simulink model "P702_NI_SoftECU"  (R2019a)
settings: Solver=ode1  StartTime=0.0  StopTime=Inf  FixedStep=0.001  RelTol=1e-3  EnableMultiTasking=on
PreLoadFcn:
  | run '.\VeriStand_BlockSet\NIVeriStandAddPaths.m'
undefined symbols (not defined in the file or in its folder): magnitude
libraries: simulink x83, simulink_extras x1
(part 72 of 76)

== system P702_NI_SoftECU/Output/Subsystem1/CAN_Signal/GWM/Other_GWMTx/Climate_Cntrl_Data_2_FD1 ==
  in_port : Inport
  ApaSwtch_D_RqDrv : Terminator
  ApaSwtch_No_Cnt : Terminator
  CabnAmb_Te_Actl : Terminator
  CamraDefog_B_Actl : Terminator
  ClimtThrmlLoad_No_Actl : Terminator
  EcoMde_D_RqDrv : Terminator
  HvacAir_Flw_Est : Terminator
  HvacBlwrFront_D_Stat : Terminator
  HvacBlwrRear_D_Stat : Terminator
  HvacRec_Pc_Est : Terminator
  HvacRemoteStrt_N_Rq : Terminator
  TwHlGrdAsst_B_RqTrn : Terminator
  bus_selector : BusSelector  OutputSignals=ApaSwtch_D_RqDrv,ApaSwtch_No_Cnt,CabnAmb_Te_Actl,CamraDefog_B_Actl,ClimtThrmlLoad_No_Actl,EcoMde_D_RqDrv,HvacAir_Flw_Est,HvacBlwrFront_D_Stat,HvacBlwrRear_D_Stat,HvacRec_Pc_Est,HvacRemoteStrt_N_Rq,TwHlGrdAsst_B_RqTrn
  wires:
  in_port/1 -> bus_selector/1  "Subsystem1"
  bus_selector/1 -> ApaSwtch_D_RqDrv/1  "<ApaSwtch_D_RqDrv>"
  bus_selector/2 -> ApaSwtch_No_Cnt/1  "<ApaSwtch_No_Cnt>"
  bus_selector/3 -> CabnAmb_Te_Actl/1  "<CabnAmb_Te_Actl>"
  bus_selector/4 -> CamraDefog_B_Actl/1  "<CamraDefog_B_Actl>"
  bus_selector/5 -> ClimtThrmlLoad_No_Actl/1  "<ClimtThrmlLoad_No_Actl>"
  bus_selector/6 -> EcoMde_D_RqDrv/1  "<EcoMde_D_RqDrv>"
  bus_selector/7 -> HvacAir_Flw_Est/1  "<HvacAir_Flw_Est>"
  bus_selector/8 -> HvacBlwrFront_D_Stat/1  "<HvacBlwrFront_D_Stat>"
  bus_selector/9 -> HvacBlwrRear_D_Stat/1  "<HvacBlwrRear_D_Stat>"
  bus_selector/10 -> HvacRec_Pc_Est/1  "<HvacRec_Pc_Est>"
  bus_selector/11 -> HvacRemoteStrt_N_Rq/1  "<HvacRemoteStrt_N_Rq>"
  bus_selector/12 -> TwHlGrdAsst_B_RqTrn/1  "<TwHlGrdAsst_B_RqTrn>"

== system P702_NI_SoftECU/Output/Subsystem1/CAN_Signal/GWM/Other_GWMTx/Climate_Control_Data_FD1 ==
  in_port : Inport
  AutoHoldSwtch_D_Stat : Terminator
  CamraFrntBttn_D_Stat : Terminator
  CamraRearBttn_D_Stat : Terminator
  DrvSlipCtlMde_B_Rq : Terminator
  EcoInhbt_B_RqHvac : Terminator
  GlvBoxRleas_No_Actl : Terminator
  LpdbAuxBlwr_B_Rq : Terminator
  LpdbDfrstFlOn_B_Rq : Terminator
  LpdbDfrstFrOn_B_Rq : Terminator
  LpdbDfrstRearOn_B_Rq : Terminator
  LpdbHeatWiprPrk_B_Rq : Terminator
  LpdbPtc1_B_Rq : Terminator
  LpdbPtc2_B_Rq : Terminator
  LpdbPtc3_B_Rq : Terminator
  MirrorHeatOn_B_Rq : Terminator
  Outside_Air_Temp_Stat : Terminator
  PrkAidSwtch_D_RqDrv : Terminator
  PrkAidSwtch_No_Cnt : Terminator
  Remote_Start_QuietMode : Terminator
  SteWhlHeat_D_Rq : Terminator
  TrailCtlSwtch_B_Stat : Terminator
  bus_selector : BusSelector  OutputSignals=AutoHoldSwtch_D_Stat,CamraFrntBttn_D_Stat,CamraRearBttn_D_Stat,DrvSlipCtlMde_B_Rq,EcoInhbt_B_RqHvac,GlvBoxRleas_No_Actl,LpdbAuxBlwr_B_Rq,LpdbDfrstFlOn_B_Rq,LpdbDfrstFrOn_B_Rq,LpdbDfrstRearOn_B_Rq,LpdbHeatWiprPrk_B_Rq,LpdbPtc1_B_Rq,LpdbPtc2_B_Rq,LpdbPtc3_B_Rq,MirrorHeatOn_B_Rq,Outside_Air_Temp_Stat,PrkAidSwtch_D_RqDrv,PrkAidSwtch_No_Cnt,Remote_Start_QuietMode,SteWhlHeat_D_Rq,TrailCtlSwtch_B_Stat
  wires:
  in_port/1 -> bus_selector/1  "Subsystem1"
  bus_selector/1 -> AutoHoldSwtch_D_Stat/1  "<AutoHoldSwtch_D_Stat>"
  bus_selector/2 -> CamraFrntBttn_D_Stat/1  "<CamraFrntBttn_D_Stat>"
  bus_selector/3 -> CamraRearBttn_D_Stat/1  "<CamraRearBttn_D_Stat>"
  bus_selector/4 -> DrvSlipCtlMde_B_Rq/1  "<DrvSlipCtlMde_B_Rq>"
  bus_selector/5 -> EcoInhbt_B_RqHvac/1  "<EcoInhbt_B_RqHvac>"
  bus_selector/6 -> GlvBoxRleas_No_Actl/1  "<GlvBoxRleas_No_Actl>"
  bus_selector/7 -> LpdbAuxBlwr_B_Rq/1  "<LpdbAuxBlwr_B_Rq>"
  bus_selector/8 -> LpdbDfrstFlOn_B_Rq/1  "<LpdbDfrstFlOn_B_Rq>"
  bus_selector/9 -> LpdbDfrstFrOn_B_Rq/1  "<LpdbDfrstFrOn_B_Rq>"
  bus_selector/10 -> LpdbDfrstRearOn_B_Rq/1  "<LpdbDfrstRearOn_B_Rq>"
  bus_selector/11 -> LpdbHeatWiprPrk_B_Rq/1  "<LpdbHeatWiprPrk_B_Rq>"
  bus_selector/12 -> LpdbPtc1_B_Rq/1  "<LpdbPtc1_B_Rq>"
  bus_selector/13 -> LpdbPtc2_B_Rq/1  "<LpdbPtc2_B_Rq>"
  bus_selector/14 -> LpdbPtc3_B_Rq/1  "<LpdbPtc3_B_Rq>"
  bus_selector/15 -> MirrorHeatOn_B_Rq/1  "<MirrorHeatOn_B_Rq>"
  bus_selector/16 -> Outside_Air_Temp_Stat/1  "<Outside_Air_Temp_Stat>"
  bus_selector/17 -> PrkAidSwtch_D_RqDrv/1  "<PrkAidSwtch_D_RqDrv>"
  bus_selector/18 -> PrkAidSwtch_No_Cnt/1  "<PrkAidSwtch_No_Cnt>"
  bus_selector/19 -> Remote_Start_QuietMode/1  "<Remote_Start_QuietMode>"
  bus_selector/20 -> SteWhlHeat_D_Rq/1  "<SteWhlHeat_D_Rq>"
  bus_selector/21 -> TrailCtlSwtch_B_Stat/1  "<TrailCtlSwtch_B_Stat>"

== system P702_NI_SoftECU/Output/Subsystem1/CAN_Signal/GWM/Other_GWMTx/Cluster_Info1_FD1 ==
  in_port : Inport
  AccDeny_B_RqIpc : Terminator
  AccEnbl_B_RqDrv : Terminator
  BulbChkActv_B_Stat : Terminator
  DrvPerfMde_D_Rq : Terminator
  DrvSlipCtlMde_B_Rq2 : Terminator
  DrvSlipCtlMde_D_Rq : Terminator
  EmgcyCallAsstMykey_Rq : Terminator
  EngIdlShutDown_B_RqDrv : Terminator
  EngOilLife_B_RqReset : Terminator
  Fda_B_Stat : Terminator
  FrostWarn_D_Stat : Terminator
  HsaMde_D_Rq : Terminator
  KeyTypeChngMykey_D_Rq : Terminator
  LscmbbStat_B_Actl : Terminator
  ManRgen_D_Rq : Terminator
  MetricActvTe_B_Actl : Terminator
  MetricActv_B_Actl : Terminator
  NtrlTowMdeEnbl_B_RqDrv : Terminator
  OdometerMasterValue : Terminator
  ParkDetect_Stat : Terminator
  Power_Liftgate_Mode_Cmd : Terminator
  PrkLckCtlEnbl_D_RqIpc : Terminator
  PtDrvMde_D_Rq : Terminator
  ReducedGuard_D_Rq : Terminator
  StopStrtDrvMde_D_RqMnu : Terminator
  TRAILER_BRAKE_CONFIG : Terminator
  TRLR_SWAY_CONFIG_CMD : Terminator
  TrlrBrkMde_D_Rq : Terminator
  bus_selector : BusSelector  OutputSignals=AccDeny_B_RqIpc,AccEnbl_B_RqDrv,BulbChkActv_B_Stat,DrvPerfMde_D_Rq,DrvSlipCtlMde_B_Rq2,DrvSlipCtlMde_D_Rq,EmgcyCallAsstMykey_Rq,EngIdlShutDown_B_RqDrv,EngOilLife_B_RqReset,Fda_B_Stat,FrostWarn_D_Stat,HsaMde_D_Rq,KeyTypeChngMykey_D_Rq,LscmbbStat_B_Actl,ManRgen_D_Rq,MetricActvTe_B_Actl,MetricActv_B_Actl,NtrlTowMdeEnbl_B_RqDrv,OdometerMasterValue,ParkDetect_Stat,Power_Liftgate_Mode_Cmd,PrkLckCtlEnbl_D_RqIpc,PtDrvMde_D_Rq,ReducedGuard_D_Rq,StopStrtDrvMde_D_RqMnu,TRAILER_BRAKE_CONFIG,TRLR_SWAY_CONFIG_CMD,TrlrBrkMde_D_Rq,ePRNDL_MODE
  ePRNDL_MODE : Terminator
  wires:
  in_port/1 -> bus_selector/1  "Subsystem1"
  bus_selector/1 -> AccDeny_B_RqIpc/1  "<AccDeny_B_RqIpc>"
  bus_selector/2 -> AccEnbl_B_RqDrv/1  "<AccEnbl_B_RqDrv>"
  bus_selector/3 -> BulbChkActv_B_Stat/1  "<BulbChkActv_B_Stat>"
  bus_selector/4 -> DrvPerfMde_D_Rq/1  "<DrvPerfMde_D_Rq>"
  bus_selector/5 -> DrvSlipCtlMde_B_Rq2/1  "<DrvSlipCtlMde_B_Rq2>"
  bus_selector/6 -> DrvSlipCtlMde_D_Rq/1  "<DrvSlipCtlMde_D_Rq>"
  bus_selector/7 -> EmgcyCallAsstMykey_Rq/1  "<EmgcyCallAsstMykey_Rq>"
  bus_selector/8 -> EngIdlShutDown_B_RqDrv/1  "<EngIdlShutDown_B_RqDrv>"
  bus_selector/9 -> EngOilLife_B_RqReset/1  "<EngOilLife_B_RqReset>"
  bus_selector/10 -> Fda_B_Stat/1  "<Fda_B_Stat>"
  bus_selector/11 -> FrostWarn_D_Stat/1  "<FrostWarn_D_Stat>"
  bus_selector/12 -> HsaMde_D_Rq/1  "<HsaMde_D_Rq>"
  bus_selector/13 -> KeyTypeChngMykey_D_Rq/1  "<KeyTypeChngMykey_D_Rq>"
  bus_selector/14 -> LscmbbStat_B_Actl/1  "<LscmbbStat_B_Actl>"
  bus_selector/15 -> ManRgen_D_Rq/1  "<ManRgen_D_Rq>"
  bus_selector/16 -> MetricActvTe_B_Actl/1  "<MetricActvTe_B_Actl>"
  bus_selector/17 -> MetricActv_B_Actl/1  "<MetricActv_B_Actl>"
  bus_selector/18 -> NtrlTowMdeEnbl_B_RqDrv/1  "<NtrlTowMdeEnbl_B_RqDrv>"
  bus_selector/19 -> OdometerMasterValue/1  "<OdometerMasterValue>"
  bus_selector/20 -> ParkDetect_Stat/1  "<ParkDetect_Stat>"
  bus_selector/21 -> Power_Liftgate_Mode_Cmd/1  "<Power_Liftgate_Mode_Cmd>"
  bus_selector/22 -> PrkLckCtlEnbl_D_RqIpc/1  "<PrkLckCtlEnbl_D_RqIpc>"
  bus_selector/23 -> PtDrvMde_D_Rq/1  "<PtDrvMde_D_Rq>"
  bus_selector/24 -> ReducedGuard_D_Rq/1  "<ReducedGuard_D_Rq>"
  bus_selector/25 -> StopStrtDrvMde_D_RqMnu/1  "<StopStrtDrvMde_D_RqMnu>"
  bus_selector/26 -> TRAILER_BRAKE_CONFIG/1  "<TRAILER_BRAKE_CONFIG>"
  bus_selector/27 -> TRLR_SWAY_CONFIG_CMD/1  "<TRLR_SWAY_CONFIG_CMD>"
  bus_selector/28 -> TrlrBrkMde_D_Rq/1  "<TrlrBrkMde_D_Rq>"
  bus_selector/29 -> ePRNDL_MODE/1  "<ePRNDL_MODE>"

== system P702_NI_SoftECU/Output/Subsystem1/CAN_Signal/GWM/Other_GWMTx/Cluster_Info_3_FD1 ==
  in_port : Inport
  AutoRgen_D_Rq : Terminator
  DISPLAY_SPEED_OFFSET : Terminator
  DISPLAY_SPEED_SCALING : Terminator
  DrvSlipCtlMde_B_RqMyKey : Terminator
  FUEL_SENSOR_NUM : Terminator
  FuelLvlActvSide_No_Raw : Terminator
  FuelLvlPssvSide_No_Raw : Terminator
  FuelLvlWarn_D_Actl : Terminator
  FuelLvl_Pc_Dsply : Terminator
  FuelSecndActv_B_Actl : Terminator
  OdoTripRx_B_Actl : Terminator
  Veh_V_CompLimMx : Terminator
  W2S_LAMP_OK : Terminator
  bus_selector : BusSelector  OutputSignals=AutoRgen_D_Rq,DISPLAY_SPEED_OFFSET,DISPLAY_SPEED_SCALING,DrvSlipCtlMde_B_RqMyKey,FUEL_SENSOR_NUM,FuelLvlActvSide_No_Raw,FuelLvlPssvSide_No_Raw,FuelLvlWarn_D_Actl,FuelLvl_Pc_Dsply,FuelSecndActv_B_Actl,OdoTripRx_B_Actl,Veh_V_CompLimMx,W2S_LAMP_OK
  wires:
  in_port/1 -> bus_selector/1  "Subsystem1"
  bus_selector/1 -> AutoRgen_D_Rq/1  "<AutoRgen_D_Rq>"
  bus_selector/2 -> DISPLAY_SPEED_OFFSET/1  "<DISPLAY_SPEED_OFFSET>"
  bus_selector/3 -> DISPLAY_SPEED_SCALING/1  "<DISPLAY_SPEED_SCALING>"
  bus_selector/4 -> DrvSlipCtlMde_B_RqMyKey/1  "<DrvSlipCtlMde_B_RqMyKey>"
  bus_selector/5 -> FUEL_SENSOR_NUM/1  "<FUEL_SENSOR_NUM>"
  bus_selector/6 -> FuelLvlActvSide_No_Raw/1  "<FuelLvlActvSide_No_Raw>"
  bus_selector/7 -> FuelLvlPssvSide_No_Raw/1  "<FuelLvlPssvSide_No_Raw>"
  bus_selector/8 -> FuelLvlWarn_D_Actl/1  "<FuelLvlWarn_D_Actl>"
  bus_selector/9 -> FuelLvl_Pc_Dsply/1  "<FuelLvl_Pc_Dsply>"
  bus_selector/10 -> FuelSecndActv_B_Actl/1  "<FuelSecndActv_B_Actl>"
  bus_selector/11 -> OdoTripRx_B_Actl/1  "<OdoTripRx_B_Actl>"
  bus_selector/12 -> Veh_V_CompLimMx/1  "<Veh_V_CompLimMx>"
  bus_selector/13 -> W2S_LAMP_OK/1  "<W2S_LAMP_OK>"

== system P702_NI_SoftECU/Output/Subsystem1/CAN_Signal/GWM/Other_GWMTx/Cluster_Lighting_Rq_FD1 ==
  in_port : Inport
  IsaOffst_D_Rq : Terminator
  SlMde_D_Rq : Terminator
  bus_selector : BusSelector  OutputSignals=IsaOffst_D_Rq,SlMde_D_Rq
  wires:
  in_port/1 -> bus_selector/1  "Subsystem1"
  bus_selector/1 -> IsaOffst_D_Rq/1  "<IsaOffst_D_Rq>"
  bus_selector/2 -> SlMde_D_Rq/1  "<SlMde_D_Rq>"

== system P702_NI_SoftECU/Output/Subsystem1/CAN_Signal/GWM/Other_GWMTx/Compressor_Req_FD1 ==
  in_port : Inport
  ClimtCoolRear_B_Rq : Terminator
  ClimtCool_D_Rq : Terminator
  ClimtDeltaLoad_Pw_Actl : Terminator
  ClimtHeatRear_D_Rq : Terminator
  ClimtHeat_D_Rq : Terminator
  ClimtPw_B_Rq : Terminator
  HtrCorePump_B_Rq : Terminator
  HvacAirCond_B_Rq : Terminator
  HvacEvap_Te_Actl : Terminator
  HvacEvap_Te_Offst : Terminator
  HvacEvap_Te_Rq : Terminator
  HvacHtrCore_Te_Rq : Terminator
  SnowPlowMde_B_Enbl : Terminator
  StopStrtDrvMde_B_RqBtn : Terminator
  WndwFrontHeat_B_Stat : Terminator
  bus_selector : BusSelector  OutputSignals=ClimtCoolRear_B_Rq,ClimtCool_D_Rq,ClimtDeltaLoad_Pw_Actl,ClimtHeatRear_D_Rq,ClimtHeat_D_Rq,ClimtPw_B_Rq,HtrCorePump_B_Rq,HvacAirCond_B_Rq,HvacEvap_Te_Actl,HvacEvap_Te_Offst,HvacEvap_Te_Rq,HvacHtrCore_Te_Rq,SnowPlowMde_B_Enbl,StopStrtDrvMde_B_RqBtn,WndwFrontHeat_B_Stat
  wires:
  in_port/1 -> bus_selector/1  "Subsystem1"
  bus_selector/1 -> ClimtCoolRear_B_Rq/1  "<ClimtCoolRear_B_Rq>"
  bus_selector/2 -> ClimtCool_D_Rq/1  "<ClimtCool_D_Rq>"
  bus_selector/3 -> ClimtDeltaLoad_Pw_Actl/1  "<ClimtDeltaLoad_Pw_Actl>"
  bus_selector/4 -> ClimtHeatRear_D_Rq/1  "<ClimtHeatRear_D_Rq>"
  bus_selector/5 -> ClimtHeat_D_Rq/1  "<ClimtHeat_D_Rq>"
  bus_selector/6 -> ClimtPw_B_Rq/1  "<ClimtPw_B_Rq>"
  bus_selector/7 -> HtrCorePump_B_Rq/1  "<HtrCorePump_B_Rq>"
  bus_selector/8 -> HvacAirCond_B_Rq/1  "<HvacAirCond_B_Rq>"
  bus_selector/9 -> HvacEvap_Te_Actl/1  "<HvacEvap_Te_Actl>"
  bus_selector/10 -> HvacEvap_Te_Offst/1  "<HvacEvap_Te_Offst>"
  bus_selector/11 -> HvacEvap_Te_Rq/1  "<HvacEvap_Te_Rq>"
  bus_selector/12 -> HvacHtrCore_Te_Rq/1  "<HvacHtrCore_Te_Rq>"
  bus_selector/13 -> SnowPlowMde_B_Enbl/1  "<SnowPlowMde_B_Enbl>"
  bus_selector/14 -> StopStrtDrvMde_B_RqBtn/1  "<StopStrtDrvMde_B_RqBtn>"
  bus_selector/15 -> WndwFrontHeat_B_Stat/1  "<WndwFrontHeat_B_Stat>"

== system P702_NI_SoftECU/Output/Subsystem1/CAN_Signal/GWM/Other_GWMTx/CruiseCtrl_Strg_Data_FD1 ==
  in_port : Inport
  AccButtnGapDecPress2 : Terminator
  AccButtnGapIncPress2 : Terminator
  AccButtnGpTogglePress2 : Terminator
  ActvFrontSteLck_D_Stat : Terminator
  ActvFrontSteMsgTxt_D_Rq : Terminator
  AslButtnOnOffCnclPres2 : Terminator
  AslButtnOnOffPress2 : Terminator
  CcAslButtnCnclPress2 : Terminator
  CcAslButtnCnclResPres2 : Terminator
  CcAslButtnDeny_B_Actl2 : Terminator
  CcAslButtnIndxDecPres2 : Terminator
  CcAslButtnIndxIncPres2 : Terminator
  CcAslButtnOffCnclPres2 : Terminator
  CcAslButtnOnOffCncl2 : Terminator
  CcAslButtnOnPress2 : Terminator
  CcAslButtnResDecPress2 : Terminator
  CcAslButtnResIncPress2 : Terminator
  CcAslButtnSetDecPress2 : Terminator
  CcAslButtnSetIncPress2 : Terminator
  CcAslButtnSetPress2 : Terminator
  CcAsllButtnResPress2 : Terminator
  CcButtnOffPress2 : Terminator
  CcButtnOnOffCnclPress2 : Terminator
  CcButtnOnOffPress2 : Terminator
  CcButtnOnPress2 : Terminator
  SelDrvMdeAdptSte_D_Stat : Terminator
  TjaButtnOnOffPress2 : Terminator
  bus_selector : BusSelector  OutputSignals=AccButtnGapDecPress2,AccButtnGapIncPress2,AccButtnGpTogglePress2,ActvFrontSteLck_D_Stat,ActvFrontSteMsgTxt_D_Rq,AslButtnOnOffCnclPres2,AslButtnOnOffPress2,CcAslButtnCnclPress2,CcAslButtnCnclResPres2,CcAslButtnDeny_B_Actl2,CcAslButtnIndxDecPres2,CcAslButtnIndxIncPres2,CcAslButtnOffCnclPres2,CcAslButtnOnOffCncl2,CcAslButtnOnPress2,CcAslButtnResDecPress2,CcAslButtnResIncPress2,CcAslButtnSetDecPress2,CcAslButtnSetIncPress2,CcAslButtnSetPress2,CcAsllButtnResPress2,CcButtnOffPress2,CcButtnOnOffCnclPress2,CcButtnOnOffPress2,CcButtnOnPress2,SelDrvMdeAdptSte_D_Stat,TjaButtnOnOffPress2
  wires:
  in_port/1 -> bus_selector/1  "Subsystem1"
  bus_selector/1 -> AccButtnGapDecPress2/1  "<AccButtnGapDecPress2>"
  bus_selector/2 -> AccButtnGapIncPress2/1  "<AccButtnGapIncPress2>"
  bus_selector/3 -> AccButtnGpTogglePress2/1  "<AccButtnGpTogglePress2>"
  bus_selector/4 -> ActvFrontSteLck_D_Stat/1  "<ActvFrontSteLck_D_Stat>"
  bus_selector/5 -> ActvFrontSteMsgTxt_D_Rq/1  "<ActvFrontSteMsgTxt_D_Rq>"
  bus_selector/6 -> AslButtnOnOffCnclPres2/1  "<AslButtnOnOffCnclPres2>"
  bus_selector/7 -> AslButtnOnOffPress2/1  "<AslButtnOnOffPress2>"
  bus_selector/8 -> CcAslButtnCnclPress2/1  "<CcAslButtnCnclPress2>"
  bus_selector/9 -> CcAslButtnCnclResPres2/1  "<CcAslButtnCnclResPres2>"
  bus_selector/10 -> CcAslButtnDeny_B_Actl2/1  "<CcAslButtnDeny_B_Actl2>"
  bus_selector/11 -> CcAslButtnIndxDecPres2/1  "<CcAslButtnIndxDecPres2>"
  bus_selector/12 -> CcAslButtnIndxIncPres2/1  "<CcAslButtnIndxIncPres2>"
  bus_selector/13 -> CcAslButtnOffCnclPres2/1  "<CcAslButtnOffCnclPres2>"
  bus_selector/14 -> CcAslButtnOnOffCncl2/1  "<CcAslButtnOnOffCncl2>"
  bus_selector/15 -> CcAslButtnOnPress2/1  "<CcAslButtnOnPress2>"
  bus_selector/16 -> CcAslButtnResDecPress2/1  "<CcAslButtnResDecPress2>"
  bus_selector/17 -> CcAslButtnResIncPress2/1  "<CcAslButtnResIncPress2>"
  bus_selector/18 -> CcAslButtnSetDecPress2/1  "<CcAslButtnSetDecPress2>"
  bus_selector/19 -> CcAslButtnSetIncPress2/1  "<CcAslButtnSetIncPress2>"
  bus_selector/20 -> CcAslButtnSetPress2/1  "<CcAslButtnSetPress2>"
  bus_selector/21 -> CcAsllButtnResPress2/1  "<CcAsllButtnResPress2>"
  bus_selector/22 -> CcButtnOffPress2/1  "<CcButtnOffPress2>"
  bus_selector/23 -> CcButtnOnOffCnclPress2/1  "<CcButtnOnOffCnclPress2>"
  bus_selector/24 -> CcButtnOnOffPress2/1  "<CcButtnOnOffPress2>"
  bus_selector/25 -> CcButtnOnPress2/1  "<CcButtnOnPress2>"
  bus_selector/26 -> SelDrvMdeAdptSte_D_Stat/1  "<SelDrvMdeAdptSte_D_Stat>"
  bus_selector/27 -> TjaButtnOnOffPress2/1  "<TjaButtnOnOffPress2>"

== system P702_NI_SoftECU/Output/Subsystem1/CAN_Signal/GWM/Other_GWMTx/DCACA_Data1_FD1 ==
  in_port : Inport
  CoolFanDcac_D_Rq : Terminator
  DcacClntFlw_D_Rq : Terminator
  DcacPlugPrsnt_B_Stat : Terminator
  DcacRdy_D_Stat : Terminator
  bus_selector : BusSelector  OutputSignals=CoolFanDcac_D_Rq,DcacClntFlw_D_Rq,DcacPlugPrsnt_B_Stat,DcacRdy_D_Stat
  wires:
  in_port/1 -> bus_selector/1  "Subsystem1"
  bus_selector/1 -> CoolFanDcac_D_Rq/1  "<CoolFanDcac_D_Rq>"
  bus_selector/2 -> DcacClntFlw_D_Rq/1  "<DcacClntFlw_D_Rq>"
  bus_selector/3 -> DcacPlugPrsnt_B_Stat/1  "<DcacPlugPrsnt_B_Stat>"
  bus_selector/4 -> DcacRdy_D_Stat/1  "<DcacRdy_D_Stat>"

== system P702_NI_SoftECU/Output/Subsystem1/CAN_Signal/GWM/Other_GWMTx/DCACA_Data2_FD1 ==
  in_port : Inport
  DcacIn_I_Actl : Terminator
  DcacIn_U_Actl : Terminator
  Dcac_Te_Actl : Terminator
  bus_selector : BusSelector  OutputSignals=DcacIn_I_Actl,DcacIn_U_Actl,Dcac_Te_Actl
  wires:
  in_port/1 -> bus_selector/1  "Subsystem1"
  bus_selector/1 -> DcacIn_I_Actl/1  "<DcacIn_I_Actl>"
  bus_selector/2 -> DcacIn_U_Actl/1  "<DcacIn_U_Actl>"
  bus_selector/3 -> Dcac_Te_Actl/1  "<Dcac_Te_Actl>"

== system P702_NI_SoftECU/Output/Subsystem1/CAN_Signal/GWM/Other_GWMTx/DCACA_Data3_FD1 ==
  in_port : Inport
  DcacIn_Pw_Mx : Terminator
  DcacOut1_Pw_Actl : Terminator
  DcacOut2_Pw_Actl : Terminator
  DcacOut_Pw_Mx : Terminator
  bus_selector : BusSelector  OutputSignals=DcacIn_Pw_Mx,DcacOut1_Pw_Actl,DcacOut2_Pw_Actl,DcacOut_Pw_Mx
  wires:
  in_port/1 -> bus_selector/1  "Subsystem1"
  bus_selector/1 -> DcacIn_Pw_Mx/1  "<DcacIn_Pw_Mx>"
  bus_selector/2 -> DcacOut1_Pw_Actl/1  "<DcacOut1_Pw_Actl>"
  bus_selector/3 -> DcacOut2_Pw_Actl/1  "<DcacOut2_Pw_Actl>"
  bus_selector/4 -> DcacOut_Pw_Mx/1  "<DcacOut_Pw_Mx>"

== system P702_NI_SoftECU/Output/Subsystem1/CAN_Signal/GWM/Other_GWMTx/DifferentialCtrlData_1_FD1 ==
  in_port : Inport
  RearDiffLck_Tq_Actl2 : Terminator
  bus_selector : BusSelector  OutputSignals=RearDiffLck_Tq_Actl2
  wires:
  in_port/1 -> bus_selector/1  "Subsystem1"
  bus_selector/1 -> RearDiffLck_Tq_Actl2/1  "<RearDiffLck_Tq_Actl2>"

== system P702_NI_SoftECU/Output/Subsystem1/CAN_Signal/GWM/Other_GWMTx/Driver_Dr_Stat_FD1 ==
  in_port : Inport
  BLISLEDStatDriverSide : Terminator
  ChildLckFdbckRd_B_Stat : Terminator
  ChildLckPw_D_Rq : Terminator
  ChildLckPw_N_Cnt : Terminator
  Driver_Lock_Sw_Cnt : Terminator
  Driver_Lock_Sw_Stat : Terminator
  KeyCylSwDrvDr_D_Stat : Terminator
  RollCodeDrvDrKeyCyl : Terminator
  RvrseMirrorChime_B_Rq : Terminator
  WndwDrvSide_D_Stat : Terminator
  bus_selector : BusSelector  OutputSignals=BLISLEDStatDriverSide,ChildLckFdbckRd_B_Stat,ChildLckPw_D_Rq,ChildLckPw_N_Cnt,Driver_Lock_Sw_Cnt,Driver_Lock_Sw_Stat,KeyCylSwDrvDr_D_Stat,RollCodeDrvDrKeyCyl,RvrseMirrorChime_B_Rq,WndwDrvSide_D_Stat
  wires:
  in_port/1 -> bus_selector/1  "Subsystem1"
  bus_selector/1 -> BLISLEDStatDriverSide/1  "<BLISLEDStatDriverSide>"
  bus_selector/2 -> ChildLckFdbckRd_B_Stat/1  "<ChildLckFdbckRd_B_Stat>"
  bus_selector/3 -> ChildLckPw_D_Rq/1  "<ChildLckPw_D_Rq>"
  bus_selector/4 -> ChildLckPw_N_Cnt/1  "<ChildLckPw_N_Cnt>"
  bus_selector/5 -> Driver_Lock_Sw_Cnt/1  "<Driver_Lock_Sw_Cnt>"
  bus_selector/6 -> Driver_Lock_Sw_Stat/1  "<Driver_Lock_Sw_Stat>"
  bus_selector/7 -> KeyCylSwDrvDr_D_Stat/1  "<KeyCylSwDrvDr_D_Stat>"
  bus_selector/8 -> RollCodeDrvDrKeyCyl/1  "<RollCodeDrvDrKeyCyl>"
  bus_selector/9 -> RvrseMirrorChime_B_Rq/1  "<RvrseMirrorChime_B_Rq>"
  bus_selector/10 -> WndwDrvSide_D_Stat/1  "<WndwDrvSide_D_Stat>"

== system P702_NI_SoftECU/Output/Subsystem1/CAN_Signal/GWM/Other_GWMTx/Dsp_Request_Signals11_FD1 ==
  in_port : Inport
  ApaMdeStat_D_RqDrv : Terminator
  ApaSwtch_D_RqMnu : Terminator
  CamAutoTowbarZoom : Terminator
  CamraOvrlDyn_D_Rq : Terminator
  CamraOvrlStat_D_Rq : Terminator
  CamraViewSplit_B_Rq : Terminator
  CamraZoomMan_D_Rq : Terminator
  DistanceBarSetting : Terminator
  PrkAidSwtch_D_RqMnu : Terminator
  bus_selector : BusSelector  OutputSignals=ApaMdeStat_D_RqDrv,ApaSwtch_D_RqMnu,CamAutoTowbarZoom,CamraOvrlDyn_D_Rq,CamraOvrlStat_D_Rq,CamraViewSplit_B_Rq,CamraZoomMan_D_Rq,DistanceBarSetting,PrkAidSwtch_D_RqMnu
  wires:
  in_port/1 -> bus_selector/1  "Subsystem1"
  bus_selector/1 -> ApaMdeStat_D_RqDrv/1  "<ApaMdeStat_D_RqDrv>"
  bus_selector/2 -> ApaSwtch_D_RqMnu/1  "<ApaSwtch_D_RqMnu>"
  bus_selector/3 -> CamAutoTowbarZoom/1  "<CamAutoTowbarZoom>"
  bus_selector/4 -> CamraOvrlDyn_D_Rq/1  "<CamraOvrlDyn_D_Rq>"
  bus_selector/5 -> CamraOvrlStat_D_Rq/1  "<CamraOvrlStat_D_Rq>"
  bus_selector/6 -> CamraViewSplit_B_Rq/1  "<CamraViewSplit_B_Rq>"
  bus_selector/7 -> CamraZoomMan_D_Rq/1  "<CamraZoomMan_D_Rq>"
  bus_selector/8 -> DistanceBarSetting/1  "<DistanceBarSetting>"
  bus_selector/9 -> PrkAidSwtch_D_RqMnu/1  "<PrkAidSwtch_D_RqMnu>"

== system P702_NI_SoftECU/Output/Subsystem1/CAN_Signal/GWM/Other_GWMTx/ElecHorizon_Data1_FD1 ==
  in_port : Inport
  EhData1_No_Actl : Terminator
  bus_selector : BusSelector  OutputSignals=EhData1_No_Actl
  wires:
  in_port/1 -> bus_selector/1  "Subsystem1"
  bus_selector/1 -> EhData1_No_Actl/1  "<EhData1_No_Actl>"

== system P702_NI_SoftECU/Output/Subsystem1/CAN_Signal/GWM/Other_GWMTx/ElecHorizon_Data2_FD1 ==
  in_port : Inport
  EhData2_No_Actl : Terminator
  bus_selector : BusSelector  OutputSignals=EhData2_No_Actl
  wires:
  in_port/1 -> bus_selector/1  "Subsystem1"
  bus_selector/1 -> EhData2_No_Actl/1  "<EhData2_No_Actl>"

== system P702_NI_SoftECU/Output/Subsystem1/CAN_Signal/GWM/Other_GWMTx/FourByFourSwitchData_FD1 ==
  in_port : Inport
  AwdLck_D_RqDrv : Terminator
  AwdMde_D_RqDrv : Terminator
  DrvSlipCtlMde_B_Rq3 : Terminator
  HdcSwtchPos_B_Actl : Terminator
  HybMdeSwtch_B_Rq : Terminator
  RearDiffLck_D_RqDrv : Terminator
  TrailCtlSwtch_B_Stat3 : Terminator
  bus_selector : BusSelector  OutputSignals=AwdLck_D_RqDrv,AwdMde_D_RqDrv,DrvSlipCtlMde_B_Rq3,HdcSwtchPos_B_Actl,HybMdeSwtch_B_Rq,RearDiffLck_D_RqDrv,TrailCtlSwtch_B_Stat3
  wires:
  in_port/1 -> bus_selector/1  "Subsystem1"
  bus_selector/1 -> AwdLck_D_RqDrv/1  "<AwdLck_D_RqDrv>"
  bus_selector/2 -> AwdMde_D_RqDrv/1  "<AwdMde_D_RqDrv>"
  bus_selector/3 -> DrvSlipCtlMde_B_Rq3/1  "<DrvSlipCtlMde_B_Rq3>"
  bus_selector/4 -> HdcSwtchPos_B_Actl/1  "<HdcSwtchPos_B_Actl>"
  bus_selector/5 -> HybMdeSwtch_B_Rq/1  "<HybMdeSwtch_B_Rq>"
  bus_selector/6 -> RearDiffLck_D_RqDrv/1  "<RearDiffLck_D_RqDrv>"
  bus_selector/7 -> TrailCtlSwtch_B_Stat3/1  "<TrailCtlSwtch_B_Stat3>"

== system P702_NI_SoftECU/Output/Subsystem1/CAN_Signal/GWM/Other_GWMTx/Front_Distance_Req_FD1 ==
  in_port : Inport
  FdsmTrgCntr_B_Actl : Terminator
  FdsmTrgDist_L_Actl : Terminator
  FdsmTrgLeft_B_Actl : Terminator
  FdsmTrgRight_B_Actl : Terminator
  LscmbbBaSens_D_Rq : Terminator
  LscmbbBlck_B_Actl : Terminator
  LscmbbBrkDecel_A_Rq : Terminator
  LscmbbBrkDecel_B_Enbl : Terminator
  LscmbbBrkDecel_No_Cnt : Terminator
  LscmbbBrkDecel_No_Cs : Terminator
  LscmbbBrkPrchg_D_Rq : Terminator
  LscmbbDeny_B_Actl : Terminator
  LscmbbEngTqMn_B_Rq : Terminator
  LscmbbMsgTxt_D_Rq : Terminator
  LscmbbPostEvnt_B_Dsply : Terminator
  LscmbbSrvcRqd_B_Rq : Terminator
  WndwFrontHeat_B_Rq : Terminator
  bus_selector : BusSelector  OutputSignals=FdsmTrgCntr_B_Actl,FdsmTrgDist_L_Actl,FdsmTrgLeft_B_Actl,FdsmTrgRight_B_Actl,LscmbbBaSens_D_Rq,LscmbbBlck_B_Actl,LscmbbBrkDecel_A_Rq,LscmbbBrkDecel_B_Enbl,LscmbbBrkDecel_No_Cnt,LscmbbBrkDecel_No_Cs,LscmbbBrkPrchg_D_Rq,LscmbbDeny_B_Actl,LscmbbEngTqMn_B_Rq,LscmbbMsgTxt_D_Rq,LscmbbPostEvnt_B_Dsply,LscmbbSrvcRqd_B_Rq,WndwFrontHeat_B_Rq
  wires:
  in_port/1 -> bus_selector/1  "Subsystem1"
  bus_selector/1 -> FdsmTrgCntr_B_Actl/1  "<FdsmTrgCntr_B_Actl>"
  bus_selector/2 -> FdsmTrgDist_L_Actl/1  "<FdsmTrgDist_L_Actl>"
  bus_selector/3 -> FdsmTrgLeft_B_Actl/1  "<FdsmTrgLeft_B_Actl>"
  bus_selector/4 -> FdsmTrgRight_B_Actl/1  "<FdsmTrgRight_B_Actl>"
  bus_selector/5 -> LscmbbBaSens_D_Rq/1  "<LscmbbBaSens_D_Rq>"
  bus_selector/6 -> LscmbbBlck_B_Actl/1  "<LscmbbBlck_B_Actl>"
  bus_selector/7 -> LscmbbBrkDecel_A_Rq/1  "<LscmbbBrkDecel_A_Rq>"
  bus_selector/8 -> LscmbbBrkDecel_B_Enbl/1  "<LscmbbBrkDecel_B_Enbl>"
  bus_selector/9 -> LscmbbBrkDecel_No_Cnt/1  "<LscmbbBrkDecel_No_Cnt>"
  bus_selector/10 -> LscmbbBrkDecel_No_Cs/1  "<LscmbbBrkDecel_No_Cs>"
  bus_selector/11 -> LscmbbBrkPrchg_D_Rq/1  "<LscmbbBrkPrchg_D_Rq>"
  bus_selector/12 -> LscmbbDeny_B_Actl/1  "<LscmbbDeny_B_Actl>"
  bus_selector/13 -> LscmbbEngTqMn_B_Rq/1  "<LscmbbEngTqMn_B_Rq>"
  bus_selector/14 -> LscmbbMsgTxt_D_Rq/1  "<LscmbbMsgTxt_D_Rq>"
  bus_selector/15 -> LscmbbPostEvnt_B_Dsply/1  "<LscmbbPostEvnt_B_Dsply>"
  bus_selector/16 -> LscmbbSrvcRqd_B_Rq/1  "<LscmbbSrvcRqd_B_Rq>"
  bus_selector/17 -> WndwFrontHeat_B_Rq/1  "<WndwFrontHeat_B_Rq>"

== system P702_NI_SoftECU/Output/Subsystem1/CAN_Signal/GWM/Other_GWMTx/GGCC_Config_Mgmt_ID_1_FD1 ==
  in_port : Inport
  VehicleGGCCData : Terminator
  bus_selector : BusSelector  OutputSignals=VehicleGGCCData
  wires:
  in_port/1 -> bus_selector/1  "Subsystem1"
  bus_selector/1 -> VehicleGGCCData/1  "<VehicleGGCCData>"

== system P702_NI_SoftECU/Output/Subsystem1/CAN_Signal/GWM/Other_GWMTx/GWM_AutoSar_NetMgmt_FD1 ==
  in_port : Inport
  GWM_AutoSarNMControl : Terminator
  GWM_AutoSarNMNodeId : Terminator
  GWM_AutoSarNMReserved{1..4} (4 alike) : Terminator
  GWM_GWNMProxy : Terminator
  GWM_GWOnBoardTester : Terminator
  bus_selector : BusSelector  OutputSignals=GWM_AutoSarNMControl,GWM_AutoSarNMNodeId,GWM_AutoSarNMReserved1,GWM_AutoSarNMReserved2,GWM_AutoSarNMReserved3,GWM_AutoSarNMReserved4,GWM_GWNMProxy,GWM_GWOnBoardTester
  wires:
  in_port/1 -> bus_selector/1  "Subsystem1"
  bus_selector/1 -> GWM_AutoSarNMControl/1  "<GWM_AutoSarNMControl>"
  bus_selector/2 -> GWM_AutoSarNMNodeId/1  "<GWM_AutoSarNMNodeId>"
  bus_selector/3 -> GWM_AutoSarNMReserved1/1  "<GWM_AutoSarNMReserved1>"
  bus_selector/4 -> GWM_AutoSarNMReserved2/1  "<GWM_AutoSarNMReserved2>"
  bus_selector/5 -> GWM_AutoSarNMReserved3/1  "<GWM_AutoSarNMReserved3>"
  bus_selector/6 -> GWM_AutoSarNMReserved4/1  "<GWM_AutoSarNMReserved4>"
  bus_selector/7 -> GWM_GWNMProxy/1  "<GWM_GWNMProxy>"
  bus_selector/8 -> GWM_GWOnBoardTester/1  "<GWM_GWOnBoardTester>"

== system P702_NI_SoftECU/Output/Subsystem1/CAN_Signal/GWM/Other_GWMTx/GlobalClock_Data_FD1 ==
  in_port : Inport
  GlblClkDay_No_Actl : Terminator
  GlblClkHr_No_Actl : Terminator
  GlblClkMnte_No_Actl : Terminator
  GlblClkScnd_No_Actl : Terminator
  GlblClkYr_No_Actl : Terminator
  bus_selector : BusSelector  OutputSignals=GlblClkDay_No_Actl,GlblClkHr_No_Actl,GlblClkMnte_No_Actl,GlblClkScnd_No_Actl,GlblClkYr_No_Actl
  wires:
  in_port/1 -> bus_selector/1  "Subsystem1"
  bus_selector/1 -> GlblClkDay_No_Actl/1  "<GlblClkDay_No_Actl>"
  bus_selector/2 -> GlblClkHr_No_Actl/1  "<GlblClkHr_No_Actl>"
  bus_selector/3 -> GlblClkMnte_No_Actl/1  "<GlblClkMnte_No_Actl>"
  bus_selector/4 -> GlblClkScnd_No_Actl/1  "<GlblClkScnd_No_Actl>"
  bus_selector/5 -> GlblClkYr_No_Actl/1  "<GlblClkYr_No_Actl>"

== system P702_NI_SoftECU/Output/Subsystem1/CAN_Signal/GWM/Other_GWMTx/Global_PATS_Cntrl_Info_FD1 ==
  in_port : Inport
  bus_selector : BusSelector  OutputSignals=immoControlCmd_T1,immoControlData_T1
  immoControlCmd_T1 : Terminator
  immoControlData_T1 : Terminator
  wires:
  in_port/1 -> bus_selector/1  "Subsystem1"
  bus_selector/1 -> immoControlCmd_T1/1  "<immoControlCmd_T1>"
  bus_selector/2 -> immoControlData_T1/1  "<immoControlData_T1>"

== system P702_NI_SoftECU/Output/Subsystem1/CAN_Signal/GWM/Other_GWMTx/IPC_Infotainment_FD1 ==
  in_port : Inport
  BeltminderAudioMute : Terminator
  Chime_Source : Terminator
  HdcOn_B_Rq : Terminator
  IPC_Attn_Info_Audio : Terminator
  IPC_MyKeyVolLimit_St : Terminator
  IPC_New_Attn_Event : Terminator
  Power_Up_Chime_Modules : Terminator
  Veh_V2_Dsply : Terminator
  bus_selector : BusSelector  OutputSignals=BeltminderAudioMute,Chime_Source,HdcOn_B_Rq,IPC_Attn_Info_Audio,IPC_MyKeyVolLimit_St,IPC_New_Attn_Event,Power_Up_Chime_Modules,Veh_V2_Dsply
  wires:
  in_port/1 -> bus_selector/1  "Subsystem1"
  bus_selector/1 -> BeltminderAudioMute/1  "<BeltminderAudioMute>"
  bus_selector/2 -> Chime_Source/1  "<Chime_Source>"
  bus_selector/3 -> HdcOn_B_Rq/1  "<HdcOn_B_Rq>"
  bus_selector/4 -> IPC_Attn_Info_Audio/1  "<IPC_Attn_Info_Audio>"
  bus_selector/5 -> IPC_MyKeyVolLimit_St/1  "<IPC_MyKeyVolLimit_St>"
  bus_selector/6 -> IPC_New_Attn_Event/1  "<IPC_New_Attn_Event>"
  bus_selector/7 -> Power_Up_Chime_Modules/1  "<Power_Up_Chime_Modules>"
  bus_selector/8 -> Veh_V2_Dsply/1  "<Veh_V2_Dsply>"

== system P702_NI_SoftECU/Output/Subsystem1/CAN_Signal/GWM/Other_GWMTx/IPC_Send_Signals_2_FD1 ==
  in_port : Inport
  ElLongTerm_L_Dsply : Terminator
  ElTrip_L_Dsply : Terminator
  FuelRange_L_Dsply : Terminator
  bus_selector : BusSelector  OutputSignals=ElLongTerm_L_Dsply,ElTrip_L_Dsply,FuelRange_L_Dsply
  wires:
  in_port/1 -> bus_selector/1  "Subsystem1"
  bus_selector/1 -> ElLongTerm_L_Dsply/1  "<ElLongTerm_L_Dsply>"
  bus_selector/2 -> ElTrip_L_Dsply/1  "<ElTrip_L_Dsply>"
  bus_selector/3 -> FuelRange_L_Dsply/1  "<FuelRange_L_Dsply>"

== system P702_NI_SoftECU/Output/Subsystem1/CAN_Signal/GWM/Other_GWMTx/MHT_EV_Wakeup_FD1 ==
  in_port : Inport
  BattChlrSov_B_Rq : Terminator
  BattChrgTrgtSoC_D_Rq : Terminator
  BattTracDrvSustn_B_Rq : Terminator
  BrkAppl_D_RqPt : Terminator
  CabnEvapSovFront_B_Rq : Terminator
  CabnEvapSovRear_B_Rq : Terminator
  HeatCoreSovRear_B_Rq : Terminator
  HtrnClntFlw_D_Rq : Terminator
  HtrnCnnctPwr_B_Stat : Terminator
  HtrnDcdcDis_B_Rq : Terminator
  PtcHtr_D_Stat : Terminator
  bus_selector : BusSelector  OutputSignals=BattChlrSov_B_Rq,BattChrgTrgtSoC_D_Rq,BattTracDrvSustn_B_Rq,BrkAppl_D_RqPt,CabnEvapSovFront_B_Rq,CabnEvapSovRear_B_Rq,HeatCoreSovRear_B_Rq,HtrnClntFlw_D_Rq,HtrnCnnctPwr_B_Stat,HtrnDcdcDis_B_Rq,PtcHtr_D_Stat
  wires:
  in_port/1 -> bus_selector/1  "Subsystem1"
  bus_selector/1 -> BattChlrSov_B_Rq/1  "<BattChlrSov_B_Rq>"
  bus_selector/2 -> BattChrgTrgtSoC_D_Rq/1  "<BattChrgTrgtSoC_D_Rq>"
  bus_selector/3 -> BattTracDrvSustn_B_Rq/1  "<BattTracDrvSustn_B_Rq>"
  bus_selector/4 -> BrkAppl_D_RqPt/1  "<BrkAppl_D_RqPt>"
  bus_selector/5 -> CabnEvapSovFront_B_Rq/1  "<CabnEvapSovFront_B_Rq>"
  bus_selector/6 -> CabnEvapSovRear_B_Rq/1  "<CabnEvapSovRear_B_Rq>"
  bus_selector/7 -> HeatCoreSovRear_B_Rq/1  "<HeatCoreSovRear_B_Rq>"
  bus_selector/8 -> HtrnClntFlw_D_Rq/1  "<HtrnClntFlw_D_Rq>"
  bus_selector/9 -> HtrnCnnctPwr_B_Stat/1  "<HtrnCnnctPwr_B_Stat>"
  bus_selector/10 -> HtrnDcdcDis_B_Rq/1  "<HtrnDcdcDis_B_Rq>"
  bus_selector/11 -> PtcHtr_D_Stat/1  "<PtcHtr_D_Stat>"

== system P702_NI_SoftECU/Output/Subsystem1/CAN_Signal/GWM/Other_GWMTx/Mc_Send_Signals_2_FD1 ==
  in_port : Inport
  BttOn_B_Rq : Terminator
  Btt_L_Actl : Terminator
  EngExhMdeQuiet_D_Rq : Terminator
  EsaOn_B_Rq : Terminator
  Mc_VehLangUsrSel_St : Terminator
  Mc_VehUnitTempUsrSel_St : Terminator
  Mc_VehUntTrpCoUsrSel_St : Terminator
  SelDrvMdeDsply_B_Avail : Terminator
  SelDrvMdeTxtReset_B_Rq : Terminator
  WaitToStartLamp_D_Falt : Terminator
  bus_selector : BusSelector  OutputSignals=BttOn_B_Rq,Btt_L_Actl,EngExhMdeQuiet_D_Rq,EsaOn_B_Rq,Mc_VehLangUsrSel_St,Mc_VehUnitTempUsrSel_St,Mc_VehUntTrpCoUsrSel_St,SelDrvMdeDsply_B_Avail,SelDrvMdeTxtReset_B_Rq,WaitToStartLamp_D_Falt
  wires:
  in_port/1 -> bus_selector/1  "Subsystem1"
  bus_selector/1 -> BttOn_B_Rq/1  "<BttOn_B_Rq>"
  bus_selector/2 -> Btt_L_Actl/1  "<Btt_L_Actl>"
  bus_selector/3 -> EngExhMdeQuiet_D_Rq/1  "<EngExhMdeQuiet_D_Rq>"
  bus_selector/4 -> EsaOn_B_Rq/1  "<EsaOn_B_Rq>"
  bus_selector/5 -> Mc_VehLangUsrSel_St/1  "<Mc_VehLangUsrSel_St>"
  bus_selector/6 -> Mc_VehUnitTempUsrSel_St/1  "<Mc_VehUnitTempUsrSel_St>"
  bus_selector/7 -> Mc_VehUntTrpCoUsrSel_St/1  "<Mc_VehUntTrpCoUsrSel_St>"
  bus_selector/8 -> SelDrvMdeDsply_B_Avail/1  "<SelDrvMdeDsply_B_Avail>"
  bus_selector/9 -> SelDrvMdeTxtReset_B_Rq/1  "<SelDrvMdeTxtReset_B_Rq>"
  bus_selector/10 -> WaitToStartLamp_D_Falt/1  "<WaitToStartLamp_D_Falt>"

== system P702_NI_SoftECU/Output/Subsystem1/CAN_Signal/GWM/Other_GWMTx/ParkAid_Aud_Warn_CmdM_FD1 ==
  in_port : Inport
  Cta_D_Rq : Terminator
  PrkAidRear_D_RqDrv : Terminator
  Sod_D_Rq : Terminator
  SteEffort_D_Rq : Terminator
  bus_selector : BusSelector  OutputSignals=Cta_D_Rq,PrkAidRear_D_RqDrv,Sod_D_Rq,SteEffort_D_Rq
  wires:
  in_port/1 -> bus_selector/1  "Subsystem1"
  bus_selector/1 -> Cta_D_Rq/1  "<Cta_D_Rq>"
  bus_selector/2 -> PrkAidRear_D_RqDrv/1  "<PrkAidRear_D_RqDrv>"
  bus_selector/3 -> Sod_D_Rq/1  "<Sod_D_Rq>"
  bus_selector/4 -> SteEffort_D_Rq/1  "<SteEffort_D_Rq>"

== system P702_NI_SoftECU/Output/Subsystem1/CAN_Signal/GWM/Other_GWMTx/Pass_Dr_Stat_FD1 ==
  in_port : Inport
  BLISLEDStatPassSide : Terminator
  ChildLckFdbckRp_B_Stat : Terminator
  Memory_1_SwPsngr_Stat : Terminator
  Memory_2_SwPsngr_Stat : Terminator
  Memory_3_SwPsngr_Stat : Terminator
  Pasngr_Lock_Sw_Cnt : Terminator
  Pasngr_Lock_Sw_Stat : Terminator
  RollCode_No_ActlPdm : Terminator
  WndwPsngrSide_D_Stat : Terminator
  bus_selector : BusSelector  OutputSignals=BLISLEDStatPassSide,ChildLckFdbckRp_B_Stat,Memory_1_SwPsngr_Stat,Memory_2_SwPsngr_Stat,Memory_3_SwPsngr_Stat,Pasngr_Lock_Sw_Cnt,Pasngr_Lock_Sw_Stat,RollCode_No_ActlPdm,WndwPsngrSide_D_Stat
  wires:
  in_port/1 -> bus_selector/1  "Subsystem1"
  bus_selector/1 -> BLISLEDStatPassSide/1  "<BLISLEDStatPassSide>"
  bus_selector/2 -> ChildLckFdbckRp_B_Stat/1  "<ChildLckFdbckRp_B_Stat>"
  bus_selector/3 -> Memory_1_SwPsngr_Stat/1  "<Memory_1_SwPsngr_Stat>"
  bus_selector/4 -> Memory_2_SwPsngr_Stat/1  "<Memory_2_SwPsngr_Stat>"
  bus_selector/5 -> Memory_3_SwPsngr_Stat/1  "<Memory_3_SwPsngr_Stat>"
  bus_selector/6 -> Pasngr_Lock_Sw_Cnt/1  "<Pasngr_Lock_Sw_Cnt>"
  bus_selector/7 -> Pasngr_Lock_Sw_Stat/1  "<Pasngr_Lock_Sw_Stat>"
  bus_selector/8 -> RollCode_No_ActlPdm/1  "<RollCode_No_ActlPdm>"
  bus_selector/9 -> WndwPsngrSide_D_Stat/1  "<WndwPsngrSide_D_Stat>"

== system P702_NI_SoftECU/Output/Subsystem1/CAN_Signal/GWM/Other_GWMTx/Personality_APIM_Data_FD1 ==
  in_port : Inport
  CtrStkDsplyOp_D_Rq : Terminator
  CtrStkFeatConfigActl : Terminator
  CtrStkFeatNoActl : Terminator
  CtrStkPersIndex_D_Actl : Terminator
  Pers1OptIn_B_Stats : Terminator
  Pers2OptIn_B_Stats : Terminator
  Pers3OptIn_B_Stats : Terminator
  Pers4OptIn_B_Stats : Terminator
  PersStore_D_Rq : Terminator
  bus_selector : BusSelector  OutputSignals=CtrStkDsplyOp_D_Rq,CtrStkFeatConfigActl,CtrStkFeatNoActl,CtrStkPersIndex_D_Actl,Pers1OptIn_B_Stats,Pers2OptIn_B_Stats,Pers3OptIn_B_Stats,Pers4OptIn_B_Stats,PersStore_D_Rq
  wires:
  in_port/1 -> bus_selector/1  "Subsystem1"
  bus_selector/1 -> CtrStkDsplyOp_D_Rq/1  "<CtrStkDsplyOp_D_Rq>"
  bus_selector/2 -> CtrStkFeatConfigActl/1  "<CtrStkFeatConfigActl>"
  bus_selector/3 -> CtrStkFeatNoActl/1  "<CtrStkFeatNoActl>"
  bus_selector/4 -> CtrStkPersIndex_D_Actl/1  "<CtrStkPersIndex_D_Actl>"
  bus_selector/5 -> Pers1OptIn_B_Stats/1  "<Pers1OptIn_B_Stats>"
  bus_selector/6 -> Pers2OptIn_B_Stats/1  "<Pers2OptIn_B_Stats>"
  bus_selector/7 -> Pers3OptIn_B_Stats/1  "<Pers3OptIn_B_Stats>"
  bus_selector/8 -> Pers4OptIn_B_Stats/1  "<Pers4OptIn_B_Stats>"
  bus_selector/9 -> PersStore_D_Rq/1  "<PersStore_D_Rq>"

== system P702_NI_SoftECU/Output/Subsystem1/CAN_Signal/GWM/Other_GWMTx/Personality_Data_FD1 ==
  in_port : Inport
  MsgCntrDsplyOp_D_Rq : Terminator
  MsgCntrFeatConfigRq : Terminator
  MsgCntrFeatNoRq : Terminator
  MsgCntrPersIndex_D_Rq : Terminator
  bus_selector : BusSelector  OutputSignals=MsgCntrDsplyOp_D_Rq,MsgCntrFeatConfigRq,MsgCntrFeatNoRq,MsgCntrPersIndex_D_Rq
  wires:
  in_port/1 -> bus_selector/1  "Subsystem1"
  bus_selector/1 -> MsgCntrDsplyOp_D_Rq/1  "<MsgCntrDsplyOp_D_Rq>"
  bus_selector/2 -> MsgCntrFeatConfigRq/1  "<MsgCntrFeatConfigRq>"
  bus_selector/3 -> MsgCntrFeatNoRq/1  "<MsgCntrFeatNoRq>"
  bus_selector/4 -> MsgCntrPersIndex_D_Rq/1  "<MsgCntrPersIndex_D_Rq>"

== system P702_NI_SoftECU/Output/Subsystem1/CAN_Signal/GWM/Other_GWMTx/Power_Liftgate_Stat_FD1 ==
  in_port : Inport
  DrLckCnt_No_ActlTgate : Terminator
  DrTGate_D_Rq : Terminator
  DrTgateChime2_D_Rq : Terminator
  Power_Liftgate_Mode_Stt : Terminator
  PwLftgtIntSw_B_Stat : Terminator
  bus_selector : BusSelector  OutputSignals=DrLckCnt_No_ActlTgate,DrTGate_D_Rq,DrTgateChime2_D_Rq,Power_Liftgate_Mode_Stt,PwLftgtIntSw_B_Stat
  wires:
  in_port/1 -> bus_selector/1  "Subsystem1"
  bus_selector/1 -> DrLckCnt_No_ActlTgate/1  "<DrLckCnt_No_ActlTgate>"
  bus_selector/2 -> DrTGate_D_Rq/1  "<DrTGate_D_Rq>"
  bus_selector/3 -> DrTgateChime2_D_Rq/1  "<DrTgateChime2_D_Rq>"
  bus_selector/4 -> Power_Liftgate_Mode_Stt/1  "<Power_Liftgate_Mode_Stt>"
  bus_selector/5 -> PwLftgtIntSw_B_Stat/1  "<PwLftgtIntSw_B_Stat>"

== system P702_NI_SoftECU/Output/Subsystem1/CAN_Signal/GWM/Other_GWMTx/PreCond_Hev_Data1_FD1 ==
  in_port : Inport
  ChrgStat_D2_Dsply : Terminator
  bus_selector : BusSelector  OutputSignals=ChrgStat_D2_Dsply
  wires:
  in_port/1 -> bus_selector/1  "Subsystem1"
  bus_selector/1 -> ChrgStat_D2_Dsply/1  "<ChrgStat_D2_Dsply>"

== system P702_NI_SoftECU/Output/Subsystem1/CAN_Signal/GWM/Other_GWMTx/PreCond_Hev_Data2_FD1 ==
  in_port : Inport
  BattTracClntFlw_Pc_Rq : Terminator
  BattTrac_I_EstVsc : Terminator
  DrvCondTpRrDefrs_B_Rq : Terminator
  HtrnAin_UHi_Actl : Terminator
  HtrnHvilOpen_B_Actl : Terminator
  HtrnMil_D_Rq : Terminator
  HtrnOvrTeLamp_B_Dsply : Terminator
  HtrnSrvcRqd_B_Dsply : Terminator
  PreCondActv_B_Actl : Terminator
  PtWakeupDeltaT_T_Rq : Terminator
  bus_selector : BusSelector  OutputSignals=BattTracClntFlw_Pc_Rq,BattTrac_I_EstVsc,DrvCondTpRrDefrs_B_Rq,HtrnAin_UHi_Actl,HtrnHvilOpen_B_Actl,HtrnMil_D_Rq,HtrnOvrTeLamp_B_Dsply,HtrnSrvcRqd_B_Dsply,PreCondActv_B_Actl,PtWakeupDeltaT_T_Rq
  wires:
  in_port/1 -> bus_selector/1  "Subsystem1"
  bus_selector/1 -> BattTracClntFlw_Pc_Rq/1  "<BattTracClntFlw_Pc_Rq>"
  bus_selector/2 -> BattTrac_I_EstVsc/1  "<BattTrac_I_EstVsc>"
  bus_selector/3 -> DrvCondTpRrDefrs_B_Rq/1  "<DrvCondTpRrDefrs_B_Rq>"
  bus_selector/4 -> HtrnAin_UHi_Actl/1  "<HtrnAin_UHi_Actl>"
  bus_selector/5 -> HtrnHvilOpen_B_Actl/1  "<HtrnHvilOpen_B_Actl>"
  bus_selector/6 -> HtrnMil_D_Rq/1  "<HtrnMil_D_Rq>"
  bus_selector/7 -> HtrnOvrTeLamp_B_Dsply/1  "<HtrnOvrTeLamp_B_Dsply>"
  bus_selector/8 -> HtrnSrvcRqd_B_Dsply/1  "<HtrnSrvcRqd_B_Dsply>"
  bus_selector/9 -> PreCondActv_B_Actl/1  "<PreCondActv_B_Actl>"
  bus_selector/10 -> PtWakeupDeltaT_T_Rq/1  "<PtWakeupDeltaT_T_Rq>"

== system P702_NI_SoftECU/Output/Subsystem1/CAN_Signal/GWM/Other_GWMTx/Suspension_Data_FD1 ==
  in_port : Inport
  SuspClkSync_No_Rq : Terminator
  SuspFrntRight_L_Actl : Terminator
  SuspFrnt_L_Actl : Terminator
  SuspFrnt_L_Prev : Terminator
  SuspRearRight_L_Actl : Terminator
  SuspRear_L_Actl : Terminator
  SuspRear_L_Prev : Terminator
  bus_selector : BusSelector  OutputSignals=SuspClkSync_No_Rq,SuspFrntRight_L_Actl,SuspFrnt_L_Actl,SuspFrnt_L_Prev,SuspRearRight_L_Actl,SuspRear_L_Actl,SuspRear_L_Prev
  wires:
  in_port/1 -> bus_selector/1  "Subsystem1"
  bus_selector/1 -> SuspClkSync_No_Rq/1  "<SuspClkSync_No_Rq>"
  bus_selector/2 -> SuspFrntRight_L_Actl/1  "<SuspFrntRight_L_Actl>"
  bus_selector/3 -> SuspFrnt_L_Actl/1  "<SuspFrnt_L_Actl>"
  bus_selector/4 -> SuspFrnt_L_Prev/1  "<SuspFrnt_L_Prev>"
  bus_selector/5 -> SuspRearRight_L_Actl/1  "<SuspRearRight_L_Actl>"
  bus_selector/6 -> SuspRear_L_Actl/1  "<SuspRear_L_Actl>"
  bus_selector/7 -> SuspRear_L_Prev/1  "<SuspRear_L_Prev>"

== system P702_NI_SoftECU/Output/Subsystem1/CAN_Signal/GWM/Other_GWMTx/TesterPhysicalResGWM_FD1 ==
  in_port : Inport
  TesterPhysicalResGWM_F1 : Terminator
  bus_selector : BusSelector  OutputSignals=TesterPhysicalResGWM_F1
  wires:
  in_port/1 -> bus_selector/1  "Subsystem1"
  bus_selector/1 -> TesterPhysicalResGWM_F1/1  "<TesterPhysicalResGWM_F1>"

== system P702_NI_SoftECU/Output/Subsystem1/CAN_Signal/GWM/Other_GWMTx/TrailerAid_Data_FD1 ==
  in_port : Inport
  TrlBrkInitOut_D_Rq : Terminator
  TrlrAidEnbl_D_Rq : Terminator
  TrlrAidSetup_D_Rq : Terminator
  TrlrAnOffstDir_D_Mem : Terminator
  TrlrAnOffst_An_Mem : Terminator
  TrlrAxleToBmpr_L_Actl : Terminator
  TrlrBallToBmpr_L_Actl : Terminator
  TrlrId_No_Actl : Terminator
  TrlrRvrseCancl_B_Rq : Terminator
  TrlrTrgtOffst_L_Actl : Terminator
  TrlrTrgtPtrnId_No_Mem : Terminator
  TrlrTrgtToBmpr_L_Actl : Terminator
  bus_selector : BusSelector  OutputSignals=TrlBrkInitOut_D_Rq,TrlrAidEnbl_D_Rq,TrlrAidSetup_D_Rq,TrlrAnOffstDir_D_Mem,TrlrAnOffst_An_Mem,TrlrAxleToBmpr_L_Actl,TrlrBallToBmpr_L_Actl,TrlrId_No_Actl,TrlrRvrseCancl_B_Rq,TrlrTrgtOffst_L_Actl,TrlrTrgtPtrnId_No_Mem,TrlrTrgtToBmpr_L_Actl
  wires:
  in_port/1 -> bus_selector/1  "Subsystem1"
  bus_selector/1 -> TrlBrkInitOut_D_Rq/1  "<TrlBrkInitOut_D_Rq>"
  bus_selector/2 -> TrlrAidEnbl_D_Rq/1  "<TrlrAidEnbl_D_Rq>"
  bus_selector/3 -> TrlrAidSetup_D_Rq/1  "<TrlrAidSetup_D_Rq>"
  bus_selector/4 -> TrlrAnOffstDir_D_Mem/1  "<TrlrAnOffstDir_D_Mem>"
  bus_selector/5 -> TrlrAnOffst_An_Mem/1  "<TrlrAnOffst_An_Mem>"
  bus_selector/6 -> TrlrAxleToBmpr_L_Actl/1  "<TrlrAxleToBmpr_L_Actl>"
  bus_selector/7 -> TrlrBallToBmpr_L_Actl/1  "<TrlrBallToBmpr_L_Actl>"
  bus_selector/8 -> TrlrId_No_Actl/1  "<TrlrId_No_Actl>"
  bus_selector/9 -> TrlrRvrseCancl_B_Rq/1  "<TrlrRvrseCancl_B_Rq>"
  bus_selector/10 -> TrlrTrgtOffst_L_Actl/1  "<TrlrTrgtOffst_L_Actl>"
  bus_selector/11 -> TrlrTrgtPtrnId_No_Mem/1  "<TrlrTrgtPtrnId_No_Mem>"
  bus_selector/12 -> TrlrTrgtToBmpr_L_Actl/1  "<TrlrTrgtToBmpr_L_Actl>"

== system P702_NI_SoftECU/Output/Subsystem1/CAN_Signal/GWM/Other_GWMTx/TrailerAid_Stat1_FD1 ==
  in_port : Inport
  TrlrSnsId_No_Actl : Terminator
  bus_selector : BusSelector  OutputSignals=TrlrSnsId_No_Actl
  wires:
  in_port/1 -> bus_selector/1  "Subsystem1"
  bus_selector/1 -> TrlrSnsId_No_Actl/1  "<TrlrSnsId_No_Actl>"

== system P702_NI_SoftECU/Output/Subsystem1/CAN_Signal/GWM/Other_GWMTx/TrailerAid_Stat2_FD1 ==
  in_port : Inport
  TrlrHitYaw_AnRate_Actl : Terminator
  TrlrHitchYaw_An_Actl : Terminator
  TrlrHitchYaw_D_Stat : Terminator
  TrlrYawWActl_D_Qf : Terminator
  TrlrYaw_W_Actl : Terminator
  bus_selector : BusSelector  OutputSignals=TrlrHitYaw_AnRate_Actl,TrlrHitchYaw_An_Actl,TrlrHitchYaw_D_Stat,TrlrYawWActl_D_Qf,TrlrYaw_W_Actl
  wires:
  in_port/1 -> bus_selector/1  "Subsystem1"
  bus_selector/1 -> TrlrHitYaw_AnRate_Actl/1  "<TrlrHitYaw_AnRate_Actl>"
  bus_selector/2 -> TrlrHitchYaw_An_Actl/1  "<TrlrHitchYaw_An_Actl>"
  bus_selector/3 -> TrlrHitchYaw_D_Stat/1  "<TrlrHitchYaw_D_Stat>"
  bus_selector/4 -> TrlrYawWActl_D_Qf/1  "<TrlrYawWActl_D_Qf>"
  bus_selector/5 -> TrlrYaw_W_Actl/1  "<TrlrYaw_W_Actl>"

== system P702_NI_SoftECU/Output/Subsystem1/CAN_Signal/GWM/Other_GWMTx/TrailerBrakeInfo_FD1 ==
  in_port : Inport
  StopLamp_B_RqTrlrBrk : Terminator
  TrlBrkInitOut_D_Stat : Terminator
  TrlrBrkActCirct_B_Falt : Terminator
  TrlrBrkActCnnct_B_Actl : Terminator
  TrlrBrkCtl_B_Falt : Terminator
  TrlrBrkDcnnt_B_Actl : Terminator
  TrlrBrkDsply_B_Rq : Terminator
  TrlrBrkGain_No_Actl : Terminator
  TrlrBrkMde_D_Actl : Terminator
  TrlrBrkOut_No_Dsply : Terminator
  bus_selector : BusSelector  OutputSignals=StopLamp_B_RqTrlrBrk,TrlBrkInitOut_D_Stat,TrlrBrkActCirct_B_Falt,TrlrBrkActCnnct_B_Actl,TrlrBrkCtl_B_Falt,TrlrBrkDcnnt_B_Actl,TrlrBrkDsply_B_Rq,TrlrBrkGain_No_Actl,TrlrBrkMde_D_Actl,TrlrBrkOut_No_Dsply
  wires:
  in_port/1 -> bus_selector/1  "Subsystem1"
  bus_selector/1 -> StopLamp_B_RqTrlrBrk/1  "<StopLamp_B_RqTrlrBrk>"
  bus_selector/2 -> TrlBrkInitOut_D_Stat/1  "<TrlBrkInitOut_D_Stat>"
  bus_selector/3 -> TrlrBrkActCirct_B_Falt/1  "<TrlrBrkActCirct_B_Falt>"
  bus_selector/4 -> TrlrBrkActCnnct_B_Actl/1  "<TrlrBrkActCnnct_B_Actl>"
  bus_selector/5 -> TrlrBrkCtl_B_Falt/1  "<TrlrBrkCtl_B_Falt>"
  bus_selector/6 -> TrlrBrkDcnnt_B_Actl/1  "<TrlrBrkDcnnt_B_Actl>"
  bus_selector/7 -> TrlrBrkDsply_B_Rq/1  "<TrlrBrkDsply_B_Rq>"
  bus_selector/8 -> TrlrBrkGain_No_Actl/1  "<TrlrBrkGain_No_Actl>"
  bus_selector/9 -> TrlrBrkMde_D_Actl/1  "<TrlrBrkMde_D_Actl>"
  bus_selector/10 -> TrlrBrkOut_No_Dsply/1  "<TrlrBrkOut_No_Dsply>"

== system P702_NI_SoftECU/Output/Subsystem1/CAN_Signal/GWM/Other_GWMTx/TrailerInfo_2_FD1 ==
  in_port : Inport
  TrlrAidAn_URate_Actl : Terminator
  TrlrAidAn_U_Actl : Terminator
  TrlrAidCtl_U_RqDrv : Terminator
  TrlrAidSwtch_D_RqDrv : Terminator
  bus_selector : BusSelector  OutputSignals=TrlrAidAn_URate_Actl,TrlrAidAn_U_Actl,TrlrAidCtl_U_RqDrv,TrlrAidSwtch_D_RqDrv
  wires:
  in_port/1 -> bus_selector/1  "Subsystem1"
  bus_selector/1 -> TrlrAidAn_URate_Actl/1  "<TrlrAidAn_URate_Actl>"
  bus_selector/2 -> TrlrAidAn_U_Actl/1  "<TrlrAidAn_U_Actl>"
  bus_selector/3 -> TrlrAidCtl_U_RqDrv/1  "<TrlrAidCtl_U_RqDrv>"
  bus_selector/4 -> TrlrAidSwtch_D_RqDrv/1  "<TrlrAidSwtch_D_RqDrv>"

== system P702_NI_SoftECU/Output/Subsystem1/CAN_Signal/GWM/Other_GWMTx/TrailerInfo_FD1 ==
  in_port : Inport
  ParkLampTrlrOut_B_Stat : Terminator
  StopLampTrlrOut_B_Stat : Terminator
  TrlrBattChrg_D_Stat : Terminator
  TrlrLampCnnct_B_Actl : Terminator
  TrlrLampCtl_D_Stat : Terminator
  TurnLampTrlrRl_B_Stat : Terminator
  TurnLampTrlrRr_B_Stat : Terminator
  bus_selector : BusSelector  OutputSignals=ParkLampTrlrOut_B_Stat,StopLampTrlrOut_B_Stat,TrlrBattChrg_D_Stat,TrlrLampCnnct_B_Actl,TrlrLampCtl_D_Stat,TurnLampTrlrRl_B_Stat,TurnLampTrlrRr_B_Stat
  wires:
  in_port/1 -> bus_selector/1  "Subsystem1"
  bus_selector/1 -> ParkLampTrlrOut_B_Stat/1  "<ParkLampTrlrOut_B_Stat>"
  bus_selector/2 -> StopLampTrlrOut_B_Stat/1  "<StopLampTrlrOut_B_Stat>"
  bus_selector/3 -> TrlrBattChrg_D_Stat/1  "<TrlrBattChrg_D_Stat>"
  bus_selector/4 -> TrlrLampCnnct_B_Actl/1  "<TrlrLampCnnct_B_Actl>"
  bus_selector/5 -> TrlrLampCtl_D_Stat/1  "<TrlrLampCtl_D_Stat>"
  bus_selector/6 -> TurnLampTrlrRl_B_Stat/1  "<TurnLampTrlrRl_B_Stat>"
  bus_selector/7 -> TurnLampTrlrRr_B_Stat/1  "<TurnLampTrlrRr_B_Stat>"

== system P702_NI_SoftECU/Output/Subsystem1/CAN_Signal/GWM/Other_GWMTx/VeyDynamics_Data_FD1 ==
  in_port : Inport
  AdptDrvMdeChassis_D_Rq : Terminator
  AdptDrvMdePt_D_Rq : Terminator
  AirSprngRateFl_D_Rq : Terminator
  AirSprngRateFr_D_Rq : Terminator
  AirSprngRateRl_D_Rq : Terminator
  AirSprngRateRr_D_Rq : Terminator
  AirSuspMsgTxt_D_Rq : Terminator
  AirSusp_D_Stat : Terminator
  BrkPadMsgTxt_D_Rq : Terminator
  CcdMsgTxt_D_RqDsply : Terminator
  Ccd_B_Falt : Terminator
  SelDrvMdeSusp_D_Stat : Terminator
  SuspDrvMde_D_Stat : Terminator
  SuspType_B_Stat : Terminator
  SuspVLim_B_Rq : Terminator
  bus_selector : BusSelector  OutputSignals=AdptDrvMdeChassis_D_Rq,AdptDrvMdePt_D_Rq,AirSprngRateFl_D_Rq,AirSprngRateFr_D_Rq,AirSprngRateRl_D_Rq,AirSprngRateRr_D_Rq,AirSuspMsgTxt_D_Rq,AirSusp_D_Stat,BrkPadMsgTxt_D_Rq,CcdMsgTxt_D_RqDsply,Ccd_B_Falt,SelDrvMdeSusp_D_Stat,SuspDrvMde_D_Stat,SuspType_B_Stat,SuspVLim_B_Rq
  wires:
  in_port/1 -> bus_selector/1  "Subsystem1"
  bus_selector/1 -> AdptDrvMdeChassis_D_Rq/1  "<AdptDrvMdeChassis_D_Rq>"
  bus_selector/2 -> AdptDrvMdePt_D_Rq/1  "<AdptDrvMdePt_D_Rq>"
  bus_selector/3 -> AirSprngRateFl_D_Rq/1  "<AirSprngRateFl_D_Rq>"
  bus_selector/4 -> AirSprngRateFr_D_Rq/1  "<AirSprngRateFr_D_Rq>"
  bus_selector/5 -> AirSprngRateRl_D_Rq/1  "<AirSprngRateRl_D_Rq>"
  bus_selector/6 -> AirSprngRateRr_D_Rq/1  "<AirSprngRateRr_D_Rq>"
  bus_selector/7 -> AirSuspMsgTxt_D_Rq/1  "<AirSuspMsgTxt_D_Rq>"
  bus_selector/8 -> AirSusp_D_Stat/1  "<AirSusp_D_Stat>"
  bus_selector/9 -> BrkPadMsgTxt_D_Rq/1  "<BrkPadMsgTxt_D_Rq>"
  bus_selector/10 -> CcdMsgTxt_D_RqDsply/1  "<CcdMsgTxt_D_RqDsply>"
  bus_selector/11 -> Ccd_B_Falt/1  "<Ccd_B_Falt>"
  bus_selector/12 -> SelDrvMdeSusp_D_Stat/1  "<SelDrvMdeSusp_D_Stat>"
  bus_selector/13 -> SuspDrvMde_D_Stat/1  "<SuspDrvMde_D_Stat>"
  bus_selector/14 -> SuspType_B_Stat/1  "<SuspType_B_Stat>"
  bus_selector/15 -> SuspVLim_B_Rq/1  "<SuspVLim_B_Rq>"

== system P702_NI_SoftECU/Output/Subsystem1/CAN_Signal/GWM/RCM/RCMSerialNumber_FD1_454 ==
  in_port : Inport
  RCMSerialNoByte{1..8} (8 alike) : Terminator
  bus_selector : BusSelector  OutputSignals=RCMSerialNoByte1,RCMSerialNoByte2,RCMSerialNoByte3,RCMSerialNoByte4,RCMSerialNoByte5,RCMSerialNoByte6,RCMSerialNoByte7,RCMSerialNoByte8
  wires:
  in_port/1 -> bus_selector/1  "Subsystem1"
  bus_selector/1 -> RCMSerialNoByte1/1  "<RCMSerialNoByte1>"
  bus_selector/2 -> RCMSerialNoByte2/1  "<RCMSerialNoByte2>"
  bus_selector/3 -> RCMSerialNoByte3/1  "<RCMSerialNoByte3>"
  bus_selector/4 -> RCMSerialNoByte4/1  "<RCMSerialNoByte4>"
  bus_selector/5 -> RCMSerialNoByte5/1  "<RCMSerialNoByte5>"
  bus_selector/6 -> RCMSerialNoByte6/1  "<RCMSerialNoByte6>"
  bus_selector/7 -> RCMSerialNoByte7/1  "<RCMSerialNoByte7>"
  bus_selector/8 -> RCMSerialNoByte8/1  "<RCMSerialNoByte8>"
